simulink model "bio_matfunc_q_matrixt"  (R2017b)
settings: Solver=VariableStepAuto  StartTime=0.0  StopTime=10.0  RelTol=1e-3
settings Model: Creator=ktrinh  LastModifiedBy=ktrinh

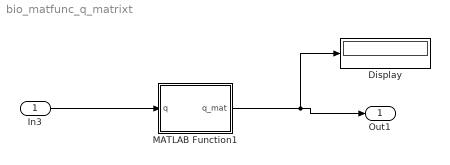
== system bio_matfunc_q_matrixt ==
  In3 : Inport  OutDataTypeStr=double  PortDimensions=4
  Display : Display
  MATLAB Function1 : MATLAB Function  TreatAsAtomicUnit=on
  Out1 : Outport
  wires:
  In3/1 -> MATLAB Function1/1(q)
  MATLAB Function1/1(q_mat) -> Display/1, Out1/1

== matlab function bio_matfunc_q_matrixt/MATLAB Function1 ==
  data: q input; q_mat output
function q_mat = q_matrix(q)
%#codegen

q_mat = [q(4) q(3) -q(2) -q(1); -q(3) q(4) q(1) -q(2); q(2) -q(1) q(4) -q(3); q(1) q(2) q(3) q(4)];
